simulink model "competition_backward_compatible"  (R2023a)
settings: Solver=ode1  StartTime=0.0  StopTime=inf  FixedStep=step_time  RelTol=1e-3  EnableMultiTasking=on
InitFcn:
  | step_time = 0.01
libraries: arduinolib x9, slpidlib x3, simulink_extras x1
settings Model: ExtModeTrigDuration=2  Creator=siche  LastModifiedBy=Jason
settings SolverCC: AutoInsertRateTranBlk=on
settings OptimizationCC: EnhancedBackFolding=on  PassReuseOutputArgsThreshold=0  MaxStackSize=64  OptimizeBlockOrder=speed  DifferentSizesBufferReuse=on  OptimizationCustomize=off
settings DebuggingCC: ParameterTunabilityLossMsg=error
settings HardwareCC: ProdBitPerInt=16  ProdBitPerPointer=16  ProdBitPerSizeT=16  ProdBitPerPtrDiffT=16  ProdLargestAtomicFloat=None  ProdWordSize=8  ProdHWDeviceType=Atmel->AVR  UseEmbeddedCoderFeatures=off
settings SFSimCC: MATLABDynamicMemAlloc=off
settings RTWCC: Description=Embedded Coder  SystemTargetFile=ert.tlc  HardwareBoard=Arduino Mega 2560  TemplateMakefile=ert_default_tmf  Toolchain=Arduino AVR
settings CodeAppCC: ForceParamTrailComments=on  OperatorAnnotations=on
settings ERTTargetCC: ERTCustomFileBanners=off  SupportContinuousTime=on  SupportNonInlinedSFcns=on  RemoveResetFunc=off  SupportVariableSizeSignals=on  ModelStepFunctionPrototypeControlCompliant=off  ExtModeTransport=3  ExtModeStaticAlloc=on  ExtModeAutomaticAllocSize=off  ExtModeStaticAllocSize=2048  ExtModeMexFile=ext_xcp  ExtModeIntrfLevel=Level2 - Open

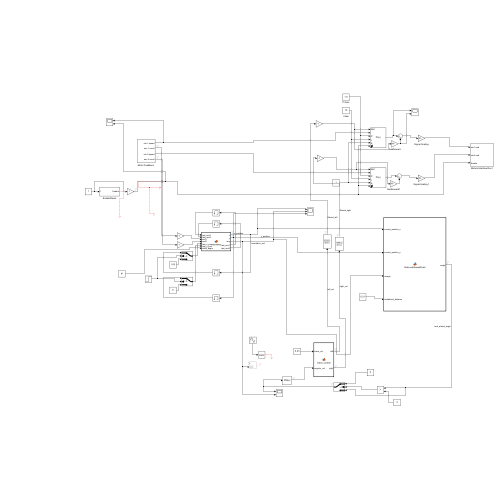
[thumbnail: Simulink's stored preview of the top-level diagram]
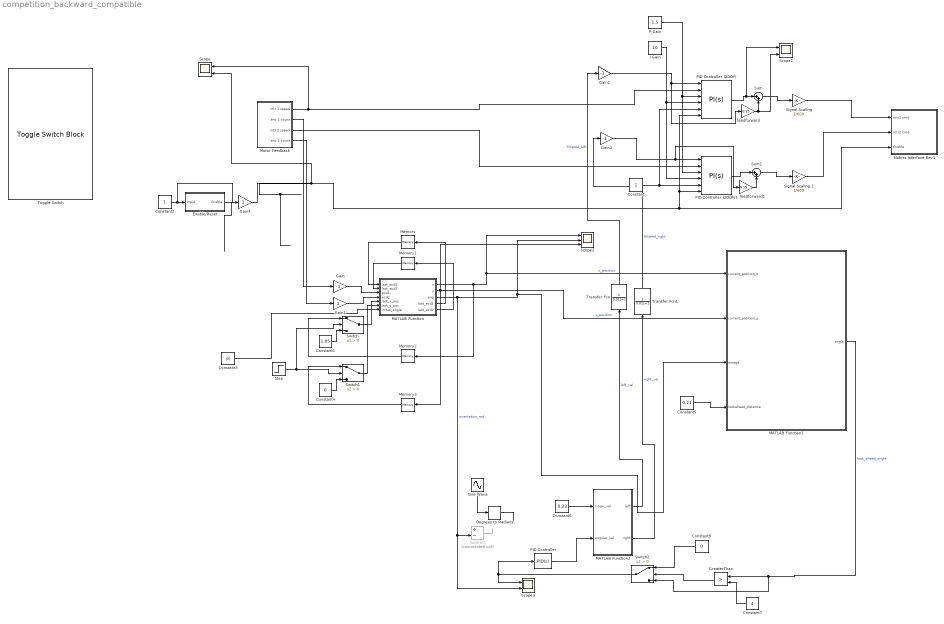
== system competition_backward_compatible ==
  Constant : Constant
  Constant1 : Constant  Value=1.05
  Constant2 : Constant
  Constant3 : Constant  Value=pi
  Constant4 : Constant  Value=0
  Constant5 : Constant  Value=0.21
  Constant6 : Constant  Value=0.23
  Constant7 : Constant  Value=4
  Constant8 : Constant  Value=0
  Degrees to Radians : simulink_extras/Transformations/Degrees to Radians
  Enable/Reset : Subsystem
  Gain : Gain  Gain=-1
  Gain1 : Gain
  Gain2 : Gain  Gain=-1
  Gain3 : Gain  Gain=-1
  Gain4 : Gain
  GreaterThan : RelationalOperator  Operator=>  OutDataTypeStr=boolean  RndMeth=Simplest  InputSameDT=off
  I Gain : Constant  Value=10
  MATLAB Function : MATLAB Function  TreatAsAtomicUnit=on
  MATLAB Function1 : MATLAB Function  TreatAsAtomicUnit=on
  MATLAB Function2 : MATLAB Function  TreatAsAtomicUnit=on
  Memory{,1..3} (4 alike) : Memory
  "Motor Feedback " : Subsystem
  Motors Interface Rev1 : Subsystem
  P Gain : Constant  Value=1.5
  PID Controller : slpidlib/PID Controller  Controller=PID  Form=Parallel  TimeDomain=Continuous-time  UseExternalTs=off  SampleTime=-1  IntegratorMethod=Forward Euler  FilterMethod=Forward Euler  ControllerParametersSource=internal  P=0.20  I=0  UseKiTs=off  D=0.02  N=100  UseFilter=on  TunerSelectOption=Transfer Function Based (PID Tuner App)  InitialConditionSource=internal  InitialConditionForIntegrator=0  InitialConditionForFilter=0  DifferentiatorICPrevScaledInput=0  ExternalReset=none  TrackingMode=off  Kt=1  LimitOutput=off  SatLimitsSource=internal  UpperSaturationLimit=inf  LowerSaturationLimit=-inf  LinearizeAsGain=on  AntiWindupMode=none  Kb=1  LimitIntegrator=off  UpperIntegratorSaturationLimit=inf  LowerIntegratorSaturationLimit=-inf  POutMin=[]  POutMax=[]  IOutMin=[]  IOutMax=[]  DOutMin=[]  DOutMax=[]  NOutMin=[]  NOutMax=[]  SumOutMin=[]  SumOutMax=[]  SaturationOutMin=[]  SaturationOutMax=[]  PParamMin=[]  PParamMax=[]  IParamMin=[]  IParamMax=[]  DParamMin=[]  DParamMax=[]  NParamMin=[]  NParamMax=[]  KbParamMin=[]  KbParamMax=[]  KtParamMin=[]  KtParamMax=[]  KbOutMin=[]  KbOutMax=[]  KtOutMin=[]  KtOutMax=[]  IntegratorOutMin=[]  IntegratorOutMax=[]  FilterOutMin=[]  FilterOutMax=[]  SumI1OutMin=[]  SumI1OutMax=[]  SumI2OutMin=[]  SumI2OutMax=[]  SumI3OutMin=[]  SumI3OutMax=[]  SumI4OutMin=[]  SumI4OutMax=[]  SumDOutMin=[]  SumDOutMax=[]  DifferentiatorOutMin=[]  DifferentiatorOutMax=[]  FilterDiffOutCoefMin=[]  FilterDiffOutCoefMax=[]  ReciprocalOutMin=[]  ReciprocalOutMax=[]  SumDenOutMin=[]  SumDenOutMax=[]  SumNumOutMin=[]  SumNumOutMax=[]  DivideOutMin=[]  DivideOutMax=[]  UdiffTsProdOutMin=[]  UdiffTsProdOutMax=[]  NTsProdOutMin=[]  NTsProdOutMax=[]  UintegralTsProdOutMin=[]  UintegralTsProdOutMax=[]  UngainTsProdOutMin=[]  UngainTsProdOutMax=[]  ClampingZeroOutDataTypeStr=Inherit: Inherit via back propagation  ClampingZeroOutMin=[]  ClampingZeroOutMax=[]  FilterDenConstantOutDataTypeStr=Inherit: Inherit via back propagation  FilterDenConstantOutMin=[]  FilterDenConstantOutMax=[]  PCopyOutDataTypeStr=Inherit: Inherit via back propagation  PCopyOutMin=[]  PCopyOutMax=[]  NCopyOutDataTypeStr=Inherit: Inherit via back propagation  NCopyOutMin=[]  NCopyOutMax=[]  IntegratorContinuousStateAttributes=''  IntegratorStateMustResolveToSignalObject=off  IntegratorRTWStateStorageClass=Auto  FilterContinuousStateAttributes=''  FilterStateMustResolveToSignalObject=off  FilterRTWStateStorageClass=Auto  ParallelPVariant=InternalParameters  IdealPVariant=Disabled  IVariant=InternalParameters  DVariant=InternalParameters  IntegratorVariant=Continuous  SatVariant=Disabled  AWVariant=Passthrough  PCopyVariant=Disabled  TRVariant=Disabled  FdbkBlocksVariant=Forward  IdealPFdbkVariant=Disabled  SatFdbkVariant=Disabled  DerivativeFilterVariant=ContFilter  NVariant=InternalParameters  NCopyVariant=Disabled  FilterICVariant=InternalICsFilter  IntegratorICVariant=InternalICs  ExternalResetVariant=Disabled  TRSumVariant=Passthrough  SumFdbkVariant=Disabled  SumVariant=Sum_PID  TsampFilterVariant=InternalTs  TsampNgainVariant=Passthrough  TsampIntegralVariant=Disabled_SignalSpec  ExternalSaturationOutDataTypeStr=Inherit: Same as second input
  PID Controller (2DOF) : slpidlib/PID Controller (2DOF)  Controller=PI  Form=Parallel  TimeDomain=Continuous-time  UseExternalTs=off  SampleTime=-1  IntegratorMethod=Forward Euler  FilterMethod=Forward Euler  ControllerParametersSource=external  P=1  I=1  UseKiTs=off  D=0  N=100  UseFilter=on  b=1  c=1  TunerSelectOption=Transfer Function Based (PID Tuner App)  InitialConditionSource=internal  InitialConditionForIntegrator=0  InitialConditionForFilter=0  DifferentiatorICPrevScaledInput=0  ExternalReset=rising  TrackingMode=off  Kt=1  LimitOutput=off  SatLimitsSource=internal  UpperSaturationLimit=inf  LowerSaturationLimit=-inf  LinearizeAsGain=on  AntiWindupMode=none  Kb=1  LimitIntegrator=off  UpperIntegratorSaturationLimit=inf  LowerIntegratorSaturationLimit=-inf  POutMin=[]  POutMax=[]  IOutMin=[]  IOutMax=[]  DOutMin=[]  DOutMax=[]  NOutMin=[]  NOutMax=[]  bOutMin=[]  bOutMax=[]  cOutMin=[]  cOutMax=[]  SumOutMin=[]  SumOutMax=[]  SaturationOutMin=[]  SaturationOutMax=[]  PParamMin=[]  PParamMax=[]  IParamMin=[]  IParamMax=[]  DParamMin=[]  DParamMax=[]  NParamMin=[]  NParamMax=[]  bParamMin=[]  bParamMax=[]  cParamMin=[]  cParamMax=[]  KbParamMin=[]  KbParamMax=[]  KtParamMin=[]  KtParamMax=[]  KbOutMin=[]  KbOutMax=[]  KtOutMin=[]  KtOutMax=[]  IntegratorOutMin=[]  IntegratorOutMax=[]  FilterOutMin=[]  FilterOutMax=[]  SumI1OutMin=[]  SumI1OutMax=[]  SumI2OutMin=[]  SumI2OutMax=[]  SumI3OutMin=[]  SumI3OutMax=[]  SumI4OutMin=[]  SumI4OutMax=[]  SumDOutMin=[]  SumDOutMax=[]  Sum1OutMin=[]  Sum1OutMax=[]  Sum2OutMin=[]  Sum2OutMax=[]  Sum3OutMin=[]  Sum3OutMax=[]  DifferentiatorOutMin=[]  DifferentiatorOutMax=[]  FilterDiffOutCoefMin=[]  FilterDiffOutCoefMax=[]  ReciprocalOutMin=[]  ReciprocalOutMax=[]  SumDenOutMin=[]  SumDenOutMax=[]  SumNumOutMin=[]  SumNumOutMax=[]  DivideOutMin=[]  DivideOutMax=[]  UdiffTsProdOutMin=[]  UdiffTsProdOutMax=[]  NTsProdOutMin=[]  NTsProdOutMax=[]  UintegralTsProdOutMin=[]  UintegralTsProdOutMax=[]  UngainTsProdOutMin=[]  UngainTsProdOutMax=[]  ClampingZeroOutDataTypeStr=Inherit: Inherit via back propagation  ClampingZeroOutMin=[]  ClampingZeroOutMax=[]  FilterDenConstantOutDataTypeStr=Inherit: Inherit via back propagation  FilterDenConstantOutMin=[]  FilterDenConstantOutMax=[]  PCopyOutDataTypeStr=Inherit: Inherit via back propagation  PCopyOutMin=[]  PCopyOutMax=[]  NCopyOutDataTypeStr=Inherit: Inherit via back propagation  NCopyOutMin=[]  NCopyOutMax=[]  IntegratorContinuousStateAttributes=''  IntegratorStateMustResolveToSignalObject=off  IntegratorRTWStateStorageClass=Auto  FilterContinuousStateAttributes=''  FilterStateMustResolveToSignalObject=off  FilterRTWStateStorageClass=Auto  ParallelPVariant=ExternalParameters  IdealPVariant=Disabled  IVariant=ExternalParameters  DVariant=Disabled  bVariant=ExternalParameters  cVariant=Disabled  IntegratorVariant=Continuous  SatVariant=Disabled  AWVariant=Passthrough  PCopyVariant=Disabled  TRVariant=Disabled  FdbkBlocksVariant=Forward  IdealPFdbkVariant=Disabled  SatFdbkVariant=Disabled  DerivativeFilterVariant=Disabled  NVariant=Disabled  NCopyVariant=Disabled_SignalSpec  FilterICVariant=Disabled  IntegratorICVariant=InternalICs  ExternalResetVariant=ExternalReset  TRSumVariant=Passthrough  SumFdbkVariant=Disabled  SumVariant=Sum_PI  TsampFilterVariant=InternalTs  TsampNgainVariant=Passthrough  TsampIntegralVariant=Disabled_SignalSpec  ExternalSaturationOutDataTypeStr=Inherit: Same as second input
  PID Controller (2DOF)1 : slpidlib/PID Controller (2DOF)  Controller=PI  Form=Parallel  TimeDomain=Continuous-time  UseExternalTs=off  SampleTime=-1  IntegratorMethod=Forward Euler  FilterMethod=Forward Euler  ControllerParametersSource=external  P=1  I=1  UseKiTs=off  D=0  N=100  UseFilter=on  b=1  c=1  TunerSelectOption=Transfer Function Based (PID Tuner App)  InitialConditionSource=internal  InitialConditionForIntegrator=0  InitialConditionForFilter=0  DifferentiatorICPrevScaledInput=0  ExternalReset=rising  TrackingMode=off  Kt=1  LimitOutput=off  SatLimitsSource=internal  UpperSaturationLimit=inf  LowerSaturationLimit=-inf  LinearizeAsGain=on  AntiWindupMode=none  Kb=1  LimitIntegrator=off  UpperIntegratorSaturationLimit=inf  LowerIntegratorSaturationLimit=-inf  POutMin=[]  POutMax=[]  IOutMin=[]  IOutMax=[]  DOutMin=[]  DOutMax=[]  NOutMin=[]  NOutMax=[]  bOutMin=[]  bOutMax=[]  cOutMin=[]  cOutMax=[]  SumOutMin=[]  SumOutMax=[]  SaturationOutMin=[]  SaturationOutMax=[]  PParamMin=[]  PParamMax=[]  IParamMin=[]  IParamMax=[]  DParamMin=[]  DParamMax=[]  NParamMin=[]  NParamMax=[]  bParamMin=[]  bParamMax=[]  cParamMin=[]  cParamMax=[]  KbParamMin=[]  KbParamMax=[]  KtParamMin=[]  KtParamMax=[]  KbOutMin=[]  KbOutMax=[]  KtOutMin=[]  KtOutMax=[]  IntegratorOutMin=[]  IntegratorOutMax=[]  FilterOutMin=[]  FilterOutMax=[]  SumI1OutMin=[]  SumI1OutMax=[]  SumI2OutMin=[]  SumI2OutMax=[]  SumI3OutMin=[]  SumI3OutMax=[]  SumI4OutMin=[]  SumI4OutMax=[]  SumDOutMin=[]  SumDOutMax=[]  Sum1OutMin=[]  Sum1OutMax=[]  Sum2OutMin=[]  Sum2OutMax=[]  Sum3OutMin=[]  Sum3OutMax=[]  DifferentiatorOutMin=[]  DifferentiatorOutMax=[]  FilterDiffOutCoefMin=[]  FilterDiffOutCoefMax=[]  ReciprocalOutMin=[]  ReciprocalOutMax=[]  SumDenOutMin=[]  SumDenOutMax=[]  SumNumOutMin=[]  SumNumOutMax=[]  DivideOutMin=[]  DivideOutMax=[]  UdiffTsProdOutMin=[]  UdiffTsProdOutMax=[]  NTsProdOutMin=[]  NTsProdOutMax=[]  UintegralTsProdOutMin=[]  UintegralTsProdOutMax=[]  UngainTsProdOutMin=[]  UngainTsProdOutMax=[]  ClampingZeroOutDataTypeStr=Inherit: Inherit via back propagation  ClampingZeroOutMin=[]  ClampingZeroOutMax=[]  FilterDenConstantOutDataTypeStr=Inherit: Inherit via back propagation  FilterDenConstantOutMin=[]  FilterDenConstantOutMax=[]  PCopyOutDataTypeStr=Inherit: Inherit via back propagation  PCopyOutMin=[]  PCopyOutMax=[]  NCopyOutDataTypeStr=Inherit: Inherit via back propagation  NCopyOutMin=[]  NCopyOutMax=[]  IntegratorContinuousStateAttributes=''  IntegratorStateMustResolveToSignalObject=off  IntegratorRTWStateStorageClass=Auto  FilterContinuousStateAttributes=''  FilterStateMustResolveToSignalObject=off  FilterRTWStateStorageClass=Auto  ParallelPVariant=ExternalParameters  IdealPVariant=Disabled  IVariant=ExternalParameters  DVariant=Disabled  bVariant=ExternalParameters  cVariant=Disabled  IntegratorVariant=Continuous  SatVariant=Disabled  AWVariant=Passthrough  PCopyVariant=Disabled  TRVariant=Disabled  FdbkBlocksVariant=Forward  IdealPFdbkVariant=Disabled  SatFdbkVariant=Disabled  DerivativeFilterVariant=Disabled  NVariant=Disabled  NCopyVariant=Disabled_SignalSpec  FilterICVariant=Disabled  IntegratorICVariant=InternalICs  ExternalResetVariant=ExternalReset  TRSumVariant=Passthrough  SumFdbkVariant=Disabled  SumVariant=Sum_PI  TsampFilterVariant=InternalTs  TsampNgainVariant=Passthrough  TsampIntegralVariant=Disabled_SignalSpec  ExternalSaturationOutDataTypeStr=Inherit: Same as second input
  Scope : Scope  NumInputPorts=2
  Scope1 : Scope  NumInputPorts=2
  Scope2 : Scope  NumInputPorts=3
  Scope3 : Scope  NumInputPorts=2
  Signal Scaling : Gain  Gain=1/600
  Signal Scaling 1 : Gain  Gain=1/600
  Sine Wave : Sin  Amplitude=5  Frequency=3  SampleTime=0
  Step : Step  Time=0.01  SampleTime=0
  Subtract : Sum  Commented=on  Inputs=+-
  Sum : Sum  Inputs=|++
  Sum1 : Sum  Inputs=|++
  Switch : Switch  Criteria=u2 > Threshold  SaturateOnIntegerOverflow=off  InputSameDT=off
  Switch1 : Switch  Criteria=u2 > Threshold  SaturateOnIntegerOverflow=off  InputSameDT=off
  Switch2 : Switch  Criteria=u2 > Threshold  SaturateOnIntegerOverflow=off  InputSameDT=off
  Toggle Switch : ToggleSwitchBlock
      settings: Values={{'Off', 'On'}, [0 1]}
  Transfer Fcn : TransferFcn  Denominator=[0.01 1]
  Transfer Fcn1 : TransferFcn  Denominator=[0.01 1]
  feedforward : Gain  Gain=0.15
  feedforward1 : Gain  Gain=0.15
  wires:
  P Gain/1 -> PID Controller (2DOF)1/3, PID Controller (2DOF)/3
  Constant/1 -> PID Controller (2DOF)1/5, PID Controller (2DOF)/5
  I Gain/1 -> PID Controller (2DOF)1/4, PID Controller (2DOF)/4
  "Motor Feedback "/1(mtr 1 speed) -> Scope/1, PID Controller (2DOF)/2
  Signal Scaling/1 -> Motors Interface Rev1/1(mtr1 cmd)
  Signal Scaling 1/1 -> Motors Interface Rev1/2(mtr2 cmd)
  "Motor Feedback "/3(mtr 2 speed) -> PID Controller (2DOF)1/2
  MATLAB Function2/1(left) -> Transfer Fcn/1  "left_vel"
  Constant2/1 -> Gain4/1, Enable/Reset/1(Input)
  PID Controller (2DOF)/1 -> Scope1/1, Sum/1
  feedforward/1 -> Scope1/2, Sum/2
  Sum/1 -> Signal Scaling/1
  "Motor Feedback "/2(enc 1 count) -> Gain/1
  "Motor Feedback "/4(enc 2 count) -> Gain1/1
  MATLAB Function/1(x) -> MATLAB Function1/1(current_position_x), Scope2/1, Memory2/1  "x_position"
  MATLAB Function/3(ang) -> Scope3/2, Subtract/2, MATLAB Function1/3(omega), Scope2/2  "orientation_rad"
  Gain/1 -> MATLAB Function/3(ecd1)
  Gain1/1 -> MATLAB Function/4(ecd2)
  MATLAB Function/4(last_ecd1) -> Memory/1
  MATLAB Function/5(last_ecd2) -> Memory1/1
  Memory1/1 -> MATLAB Function/2("last_ecd2 ")
  Memory/1 -> MATLAB Function/1("last_ecd1 ")
  Constant1/1 -> Switch/3
  Switch/1 -> MATLAB Function/5(last_x_pos)
  Memory2/1 -> Switch/1
  Memory3/1 -> Switch1/1
  Constant4/1 -> Switch1/3
  Enable/Reset/1(Enable) -> ?
  MATLAB Function/2(y) -> MATLAB Function1/2(current_position_y), Memory3/1, Scope2/3  "y_position"
  Switch1/1 -> MATLAB Function/6(last_y_pos)
  Subtract/1 -> ?
  PID Controller/1 -> MATLAB Function2/2(angular_vel)
  Constant6/1 -> MATLAB Function2/1(linear_vel)
  Gain2/1 -> feedforward/1, PID Controller (2DOF)/1
  Sum1/1 -> Signal Scaling 1/1
  feedforward1/1 -> Sum1/2
  PID Controller (2DOF)1/1 -> Sum1/1
  Gain3/1 -> feedforward1/1, PID Controller (2DOF)1/1
  MATLAB Function2/2(right) -> Transfer Fcn1/1  "right_vel"
  Sine Wave/1 -> Degrees to Radians/1
  Transfer Fcn/1 -> Gain2/1  "filtered_left"
  Transfer Fcn1/1 -> Gain3/1  "filtered_right"
  Constant3/1 -> MATLAB Function/7(initial_angle)
  Constant5/1 -> MATLAB Function1/4(lookahead_distance)
  Switch2/1 -> PID Controller/1, Scope3/1
  MATLAB Function1/1(angle) -> Switch2/3, GreaterThan/1  "look_ahead_angle"
  Constant7/1 -> GreaterThan/2
  GreaterThan/1 -> Switch2/2
  Constant8/1 -> Switch2/1
  Degrees to Radians/1 -> ?
  Step/1 -> Switch1/2, Switch/2
  Gain4/1 -> Motors Interface Rev1/3(Enable), PID Controller (2DOF)1/6, PID Controller (2DOF)/6, Scope/2

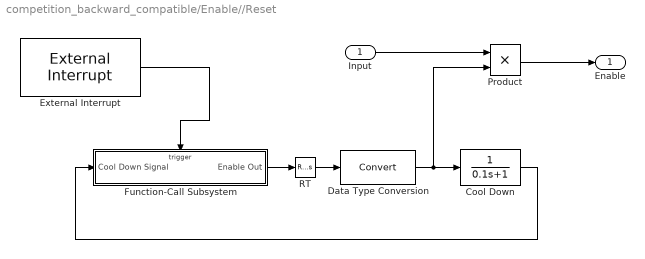
== system competition_backward_compatible/Enable//Reset ==
  Input : Inport
  Cool Down : TransferFcn  Denominator=[0.1 1]
  Data Type Conversion : DataTypeConversion  SaturateOnIntegerOverflow=off  RndMeth=Floor
  External Interrupt : arduinolib/External Interrupt  Pin=18  PullUp=on  Mode=FALLING  InterruptSimulationInput=off
  Function-Call Subsystem : Subsystem  TreatAsAtomicUnit=on
  Product : Product
  RT : RateTransition  Deterministic=off  OutPortSampleTime=step_time
  Enable : Outport
  wires:
  External Interrupt/1 -> Function-Call Subsystem/Trigger
  RT/1 -> Data Type Conversion/1
  Data Type Conversion/1 -> Product/2, Cool Down/1
  Function-Call Subsystem/1(Enable Out) -> RT/1
  Cool Down/1 -> Function-Call Subsystem/1(Cool Down Signal)
  Input/1 -> Product/1
  Product/1 -> Enable/1

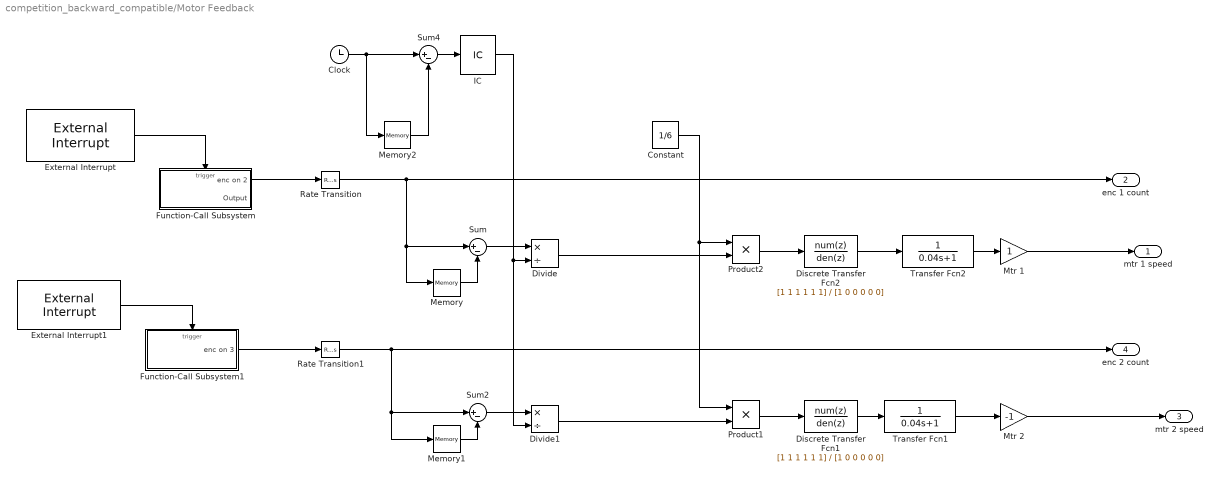
== system competition_backward_compatible/Motor Feedback  ==
  Clock : Clock
  Constant : Constant  Value=1/6
  Discrete Transfer Fcn1 : DiscreteTransferFcn  Numerator=[1 1 1 1 1 1]  Denominator=[1 0 0 0 0 0]
  Discrete Transfer Fcn2 : DiscreteTransferFcn  Numerator=[1 1 1 1 1 1]  Denominator=[1 0 0 0 0 0]
  Divide : Product  Inputs=*/
  Divide1 : Product  Inputs=*/
  External Interrupt : arduinolib/External Interrupt  Pin=2  PullUp=on  Mode=RISING  InterruptSimulationInput=off
  External Interrupt1 : arduinolib/External Interrupt  Pin=3  PullUp=on  Mode=RISING  InterruptSimulationInput=off
  Function-Call Subsystem : Subsystem  TreatAsAtomicUnit=on
  Function-Call Subsystem1 : Subsystem  TreatAsAtomicUnit=on
  IC : InitialCondition  Value=0.001
  Memory : Memory
  Memory1 : Memory
  Memory2 : Memory
  Mtr 1 : Gain
  Mtr 2 : Gain  Gain=-1
  Product1 : Product
  Product2 : Product
  Rate Transition : RateTransition  Deterministic=off  OutPortSampleTime=step_time
  Rate Transition1 : RateTransition  Deterministic=off  OutPortSampleTime=step_time
  Sum : Sum  Inputs=|+-
  Sum2 : Sum  Inputs=|+-
  Sum4 : Sum  Inputs=|+-
  Transfer Fcn1 : TransferFcn  Denominator=[0.04 1]
  Transfer Fcn2 : TransferFcn  Denominator=[0.04 1]
  mtr 1 speed : Outport
  enc 1 count : Outport  Port=2
  mtr 2 speed : Outport  Port=3
  enc 2 count : Outport  Port=4
  wires:
  IC/1 -> Divide1/2, Divide/2
  Sum4/1 -> IC/1
  Sum2/1 -> Divide1/1
  Sum/1 -> Divide/1
  Clock/1 -> Memory2/1, Sum4/1
  Memory2/1 -> Sum4/2
  Mtr 2/1 -> mtr 2 speed/1
  Mtr 1/1 -> mtr 1 speed/1
  Transfer Fcn1/1 -> Mtr 2/1
  Memory1/1 -> Sum2/2
  External Interrupt1/1 -> Function-Call Subsystem1/Trigger
  Function-Call Subsystem1/1(enc on 3) -> Rate Transition1/1
  Memory/1 -> Sum/2
  External Interrupt/1 -> Function-Call Subsystem/Trigger
  Transfer Fcn2/1 -> Mtr 1/1
  Function-Call Subsystem/1(enc on 2) -> Rate Transition/1
  Constant/1 -> Product1/1, Product2/1
  Divide/1 -> Product2/2
  Product1/1 -> Discrete Transfer Fcn1/1
  Product2/1 -> Discrete Transfer Fcn2/1
  Divide1/1 -> Product1/2
  Discrete Transfer Fcn2/1 -> Transfer Fcn2/1
  Discrete Transfer Fcn1/1 -> Transfer Fcn1/1
  Rate Transition/1 -> enc 1 count/1, Memory/1, Sum/1
  Rate Transition1/1 -> enc 2 count/1, Memory1/1, Sum2/1

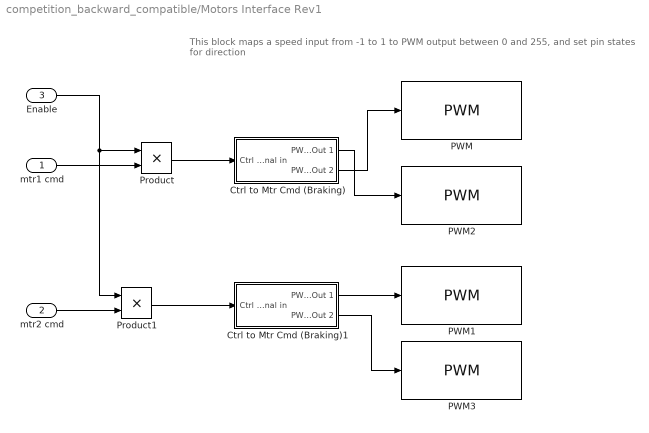
== system competition_backward_compatible/Motors Interface Rev1 ==
  note: This block maps a speed input from -1 to 1 to PWM output between 0 and 255, and set pin states for direction
  mtr1 cmd : Inport
  mtr2 cmd : Inport  Port=2
  Enable : Inport  Port=3
  Ctrl to Mtr Cmd (Braking) : Subsystem
  Ctrl to Mtr Cmd (Braking)1 : Subsystem
  PWM : arduinolib/PWM  pinNumber=6  frequencyType=Default  desiredFrequency=490.2  achievableFrequency=490.2
  PWM1 : arduinolib/PWM  pinNumber=9  frequencyType=Default  desiredFrequency=490.2  achievableFrequency=490.2
  PWM2 : arduinolib/PWM  pinNumber=7  frequencyType=Default  desiredFrequency=490.2  achievableFrequency=490.2
  PWM3 : arduinolib/PWM  pinNumber=8  frequencyType=Default  desiredFrequency=490.2  achievableFrequency=490.2
  Product : Product
  Product1 : Product
  wires:
  Ctrl to Mtr Cmd (Braking)/1(PWM Out 1) -> PWM2/1
  Ctrl to Mtr Cmd (Braking)/2(PWM Out 2) -> PWM/1
  Ctrl to Mtr Cmd (Braking)1/2(PWM Out 2) -> PWM3/1
  Ctrl to Mtr Cmd (Braking)1/1(PWM Out 1) -> PWM1/1
  Product1/1 -> Ctrl to Mtr Cmd (Braking)1/1(Ctrl Signal in)
  mtr2 cmd/1 -> Product1/2
  mtr1 cmd/1 -> Product/2
  Enable/1 -> Product/1, Product1/1
  Product/1 -> Ctrl to Mtr Cmd (Braking)/1(Ctrl Signal in)

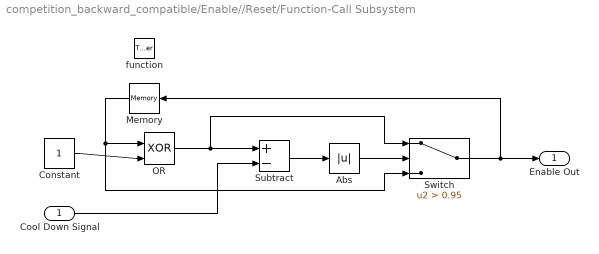
== system competition_backward_compatible/Enable//Reset/Function-Call Subsystem ==
  Cool Down Signal : Inport
  function : TriggerPort  TriggerType=function-call  VariantControl=(inherit)
  Abs : Abs  SaturateOnIntegerOverflow=off
  Constant : Constant
  Memory : Memory  InheritSampleTime=on
  OR : Logic  Operator=XOR  IconShape=distinctive  AllPortsSameDT=off  OutDataTypeStr=boolean
  Subtract : Sum  Inputs=+-
  Switch : Switch  Criteria=u2 > Threshold  Threshold=0.95  SaturateOnIntegerOverflow=off  InputSameDT=off
  Enable Out : Outport  InitialOutput=0
  wires:
  Constant/1 -> OR/2
  OR/1 -> Switch/1, Subtract/1
  Memory/1 -> Switch/3, OR/1
  Cool Down Signal/1 -> Subtract/2
  Subtract/1 -> Abs/1
  Abs/1 -> Switch/2
  Switch/1 -> Memory/1, Enable Out/1

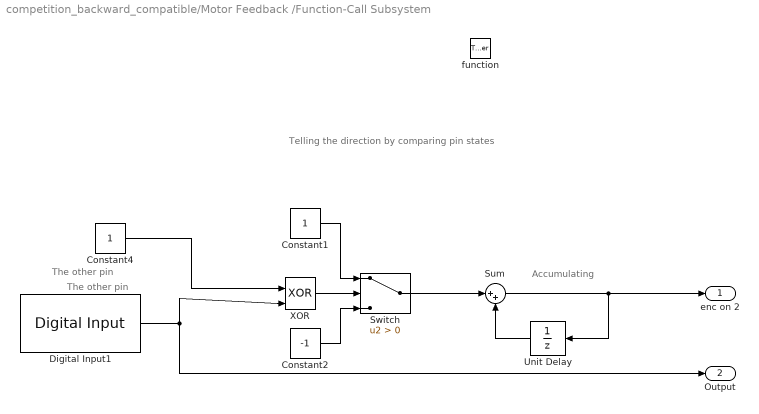
== system competition_backward_compatible/Motor Feedback /Function-Call Subsystem ==
  note: The other pin
  note: The other pin
  note: Telling the direction by comparing pin states
  note: Accumulating
  function : TriggerPort  TriggerType=function-call  VariantControl=(inherit)
  Constant1 : Constant
  Constant2 : Constant  Value=-1
  Constant4 : Constant
  Digital Input1 : arduinolib/Digital Input  pinNumber=4  mode=Input Pullup  Direction=input  SampleTime=-1  blockPlatform=arduino
  Sum : Sum  Inputs=|++
  Switch : Switch  Criteria=u2 > Threshold  SaturateOnIntegerOverflow=off  InputSameDT=off
  Unit Delay : UnitDelay  SampleTime=-1  HasFrameUpgradeWarning=on
  XOR : Logic  Operator=XOR  IconShape=distinctive  AllPortsSameDT=off  OutDataTypeStr=boolean
  enc on 2 : Outport  InitialOutput=0
  Output : Outport  Port=2  OutputWhenDisabled=reset  InitialOutput=0
  wires:
  Digital Input1/1 -> XOR/2, Output/1
  Constant4/1 -> XOR/1
  Switch/1 -> Sum/1
  XOR/1 -> Switch/2
  Constant1/1 -> Switch/1
  Constant2/1 -> Switch/3
  Unit Delay/1 -> Sum/2
  Sum/1 -> enc on 2/1, Unit Delay/1

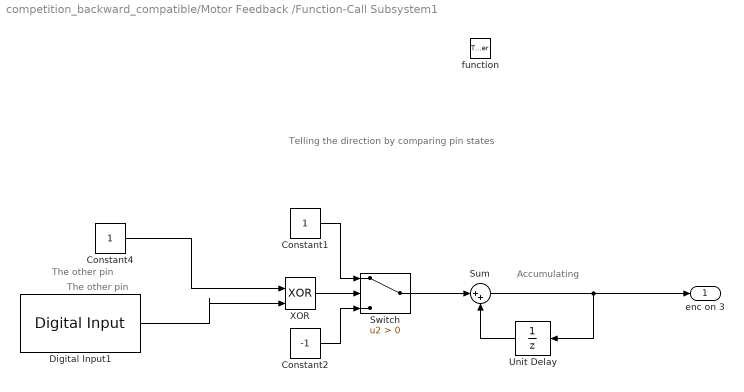
== system competition_backward_compatible/Motor Feedback /Function-Call Subsystem1 ==
  note: The other pin
  note: The other pin
  note: Telling the direction by comparing pin states
  note: Accumulating
  function : TriggerPort  TriggerType=function-call  VariantControl=(inherit)
  Constant1 : Constant
  Constant2 : Constant  Value=-1
  Constant4 : Constant
  Digital Input1 : arduinolib/Digital Input  pinNumber=5  mode=Input Pullup  Direction=input  SampleTime=-1  blockPlatform=arduino
  Sum : Sum  Inputs=|++
  Switch : Switch  Criteria=u2 > Threshold  SaturateOnIntegerOverflow=off  InputSameDT=off
  Unit Delay : UnitDelay  SampleTime=-1  HasFrameUpgradeWarning=on
  XOR : Logic  Operator=XOR  IconShape=distinctive  AllPortsSameDT=off  OutDataTypeStr=boolean
  enc on 3 : Outport  InitialOutput=0
  wires:
  Constant4/1 -> XOR/1
  Switch/1 -> Sum/1
  Digital Input1/1 -> XOR/2
  XOR/1 -> Switch/2
  Constant1/1 -> Switch/1
  Constant2/1 -> Switch/3
  Unit Delay/1 -> Sum/2
  Sum/1 -> enc on 3/1, Unit Delay/1

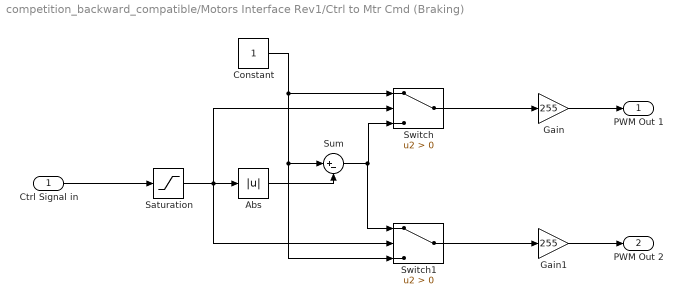
== system competition_backward_compatible/Motors Interface Rev1/Ctrl to Mtr Cmd (Braking) ==
  Ctrl Signal in : Inport
  Abs : Abs  SaturateOnIntegerOverflow=off
  Constant : Constant
  Gain : Gain  Gain=255
  Gain1 : Gain  Gain=255
  Saturation : Saturate  UpperLimit=1  LowerLimit=-1
  Sum : Sum  Inputs=|+-
  Switch : Switch  Criteria=u2 > Threshold  SaturateOnIntegerOverflow=off  InputSameDT=off
  Switch1 : Switch  Criteria=u2 > Threshold  SaturateOnIntegerOverflow=off  InputSameDT=off
  PWM Out 1 : Outport
  PWM Out 2 : Outport  Port=2
  wires:
  Gain1/1 -> PWM Out 2/1
  Gain/1 -> PWM Out 1/1
  Switch/1 -> Gain/1
  Switch1/1 -> Gain1/1
  Sum/1 -> Switch/3, Switch1/1
  Abs/1 -> Sum/2
  Ctrl Signal in/1 -> Saturation/1
  Saturation/1 -> Switch/2, Switch1/2, Abs/1
  Constant/1 -> Switch/1, Switch1/3, Sum/1

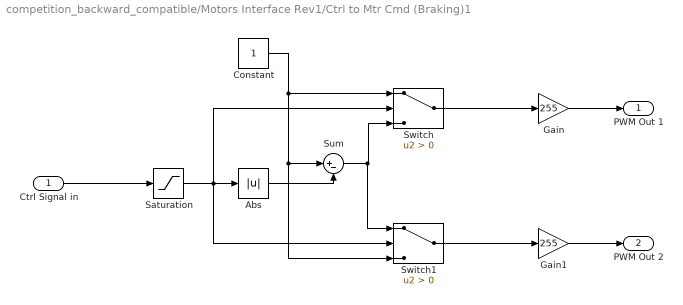
== system competition_backward_compatible/Motors Interface Rev1/Ctrl to Mtr Cmd (Braking)1 ==
  Ctrl Signal in : Inport
  Abs : Abs  SaturateOnIntegerOverflow=off
  Constant : Constant
  Gain : Gain  Gain=255
  Gain1 : Gain  Gain=255
  Saturation : Saturate  UpperLimit=1  LowerLimit=-1
  Sum : Sum  Inputs=|+-
  Switch : Switch  Criteria=u2 > Threshold  SaturateOnIntegerOverflow=off  InputSameDT=off
  Switch1 : Switch  Criteria=u2 > Threshold  SaturateOnIntegerOverflow=off  InputSameDT=off
  PWM Out 1 : Outport
  PWM Out 2 : Outport  Port=2
  wires:
  Gain1/1 -> PWM Out 2/1
  Gain/1 -> PWM Out 1/1
  Switch/1 -> Gain/1
  Switch1/1 -> Gain1/1
  Sum/1 -> Switch/3, Switch1/1
  Abs/1 -> Sum/2
  Ctrl Signal in/1 -> Saturation/1
  Saturation/1 -> Switch/2, Switch1/2, Abs/1
  Constant/1 -> Switch/1, Switch1/3, Sum/1

== matlab function competition_backward_compatible/MATLAB Function ==
  data: last_ecd1 input; last_ecd2 input; ecd1 input; x output; y output; ecd2 input; ang output; last_ecd1 output; last_ecd2 output; last_x_pos input; last_y_pos input; initial_angle input
function [x, y, ang, last_ecd1, last_ecd2] = odometry(last_ecd1, last_ecd2, ecd1, ecd2, last_x_pos, last_y_pos, initial_angle)

d_w = 0.042;
d_r = 0.158;
l_w = d_w * pi;
left_ratio = 45.607;
right_ratio = 40.286;
left_tick_to_meter = 1/301;
right_tick_to_meter = 1/256.67;

left =  (ecd1 - last_ecd1) * left_tick_to_meter;
right =  (ecd2 - last_ecd2) * right_tick_to_meter;
dist = (left + right) / 2;
ang = (ecd2 - ecd1) / (325.2) * 2 * pi + initial_angle;

last_ecd1 = ecd1;
last_ecd2 = ecd2;
x = last_x_pos + dist * cos(ang);
y = last_y_pos + dist * sin(ang);

end

== matlab function competition_backward_compatible/MATLAB Function2 ==
  data: linear_vel input; left output; angular_vel input; right output
function [left, right] = robot_control(linear_vel, angular_vel)
left = linear_vel - angular_vel;
right = linear_vel + angular_vel;
left = left*600;
right = right*600;
end

== matlab function competition_backward_compatible/MATLAB Function1 ==
  data: angle output; current_position_x input; current_position_y input; omega input; lookahead_distance input
function angle = findLookAheadPoint(current_position_x, current_position_y, omega, lookahead_distance)
%%%%%%%%%%%%% Function Definition Start Here %%%%%%%%%%%%%
    function inrange = is_in_range(x, x_min, x_max)
    
    inrange = x<=max(x_min,x_max+0.1) && x>=min(x_min-0.1,x_max);
end

function is_ahead = isPointAhead(point, current_position, omega)
% Calculate direction vectors
direction_path = [cos(omega), sin(omega)]; % direction of the path (for non-vertical lines)
direction_vehicle_to_point = point - current_position;

% Check if the point is ahead using dot product
is_ahead = dot(direction_vehicle_to_point, direction_path) > 0;
end

function [x,y]=line_circ(slope,intercpt,centerx,centery,radius)
	a=1+slope.^2;
	b=2*(slope.*(intercpt-centery)-centerx);
	c=centery.^2+centerx.^2+intercpt.^2-2*centery.*intercpt-radius.^2;

	x=zeros(2,1);
    delta = b^2-4*a*c;
    if (b^2-4*a*c > 0)
        x(1) = (-b + sqrt(delta))/(2*a);
        x(2) = (-b - sqrt(delta))/(2*a);
		y=intercpt+slope.*x;
    else
        x= [99999; 99999];
        y = [99999; 99999];
    end
end

%%%%%%%%%%%%% Function Definition End Here %%%%%%%%%%%%%
% Extract x and y coordinates of the waypoints

length_filed = 1.05
tracking_x = [length_filed+0.05,    0-0.05,     0.001-0.05,      length_filed,           length_filed+0.01]
tracking_y = [0-0.01,               0,      length_filed ,      length_filed+0.01,      0]

x =  tracking_x;
y = tracking_y;
current_position = [current_position_x, current_position_y];
% Initialize the lookahead point
angle = 100;
% Iterate through each segment in the path
for i = 1:length(x)-1
    % Calculate slope and intercept for the line segment
    if x(i+1) == x(i) % Handle vertical lines
        slope = 999999999;
    else
        slope = (y(i+1) - y(i)) / (x(i+1) - x(i));
    end
    intercept = y(i) - slope * x(i);

    % Find intersection of line segment with the circle
    [xout, yout] = line_circ(slope, intercept, current_position(1), current_position(2), lookahead_distance);

    % Check if intersection points are valid and choose the correct point
    for j = 1:2
        if xout(j) < 9900 && is_in_range(xout(j), x(i), x(i+1)) && is_in_range(yout(j), y(i), y(i+1)) && isPointAhead([xout(j), yout(j)], current_position(1:2), omega)
            angle = atan2(yout(j)-current_position(2), xout(j) - current_position(1));
            angle = angle - omega;
            angle = mod(angle, 2*pi);
            if angle > pi
                angle = angle - 2 * pi;
            end
            return; % Return the first valid lookahead point
        end
    end
end
end
